simulink model "untitled1"  (R2025b)
settings: Solver=VariableStepAuto  StartTime=0.0  StopTime=10.0  RelTol=1e-3
values from neighbouring files (symbols this model uses):
  K1 = lqr(A,B,Q,R)    [untitled.m]
settings Model: Creator=jacksonwright  LastModifiedBy=jacksonwright

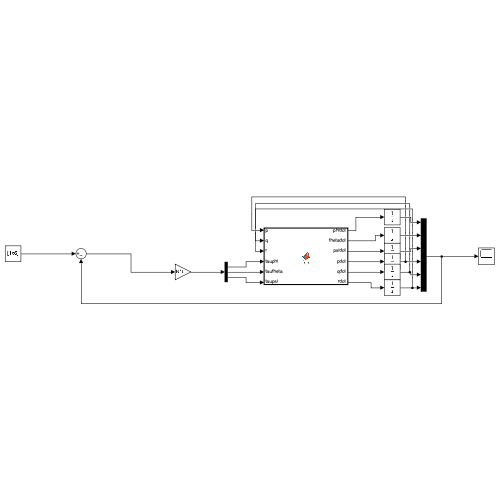
[thumbnail: Simulink's stored preview of the top-level diagram]
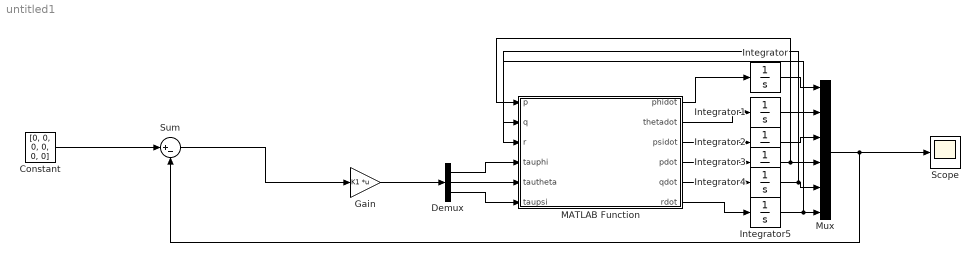
== system untitled1 ==
  Constant : Constant  Value=[0, 0, 0, 0, 0, 0]
  Demux : Demux  Outputs=3
  Gain : Gain  Gain=K1  Multiplication=Matrix(K*u)
  Integrator : Integrator  InitialCondition=0.1
  Integrator{1..5} (5 alike) : Integrator
  MATLAB Function : MATLAB Function  TreatAsAtomicUnit=on
  Mux : Mux  Inputs=6
  Scope : Scope
      settings: ActiveDisplayYMinimum=-0.16503078467277554  ActiveDisplayYMaximum=0.15659664367010984
  Sum : Sum  Inputs=|+-
  wires:
  Gain/1 -> Demux/1
  MATLAB Function/1(phidot) -> Integrator/1
  MATLAB Function/2(thetadot) -> Integrator1/1
  MATLAB Function/3(psidot) -> Integrator2/1
  MATLAB Function/4(pdot) -> Integrator3/1
  MATLAB Function/5(qdot) -> Integrator4/1
  MATLAB Function/6(rdot) -> Integrator5/1
  Sum/1 -> Gain/1
  Constant/1 -> Sum/1
  Mux/1 -> Sum/2, Scope/1
  Demux/2 -> MATLAB Function/5(tautheta)
  Demux/1 -> MATLAB Function/4(tauphi)
  Demux/3 -> MATLAB Function/6(taupsi)
  Integrator/1 -> Mux/1
  Integrator1/1 -> Mux/2
  Integrator2/1 -> Mux/3
  Integrator3/1 -> Mux/4, MATLAB Function/1(p)
  Integrator5/1 -> MATLAB Function/3(r), Mux/6
  Integrator4/1 -> MATLAB Function/2(q), Mux/5

== matlab function untitled1/MATLAB Function ==
  data: phidot output; thetadot output; psidot output; p input; q input; r input; pdot output; tauphi input; qdot output; tautheta input; rdot output; taupsi input
function [phidot, thetadot, psidot, pdot, qdot, rdot] = fcn(p, q, r, tauphi, tautheta, taupsi)

%constants
Ix = 1;
Iy = 1;
Iz = 1;

%Angular Acceleration
pdot = tauphi / Ix;
qdot = tautheta / Iy;
rdot = taupsi/ Iz;

%Angular Velocity
phidot = p;
thetadot = q;
psidot = r;
